simulink library "PhaseCurrentsChecker"  (R2016b)
settings: Solver=VariableStepAuto  StartTime=0.0  StopTime=10.0  RelTol=1e-3
undefined symbols (not defined in the file): maxPhasePeakCurrent
settings Model: Creator=Nathan  LastModifiedBy=march

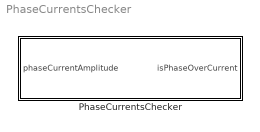
== system PhaseCurrentsChecker ==
  PhaseCurrentsChecker : Subsystem

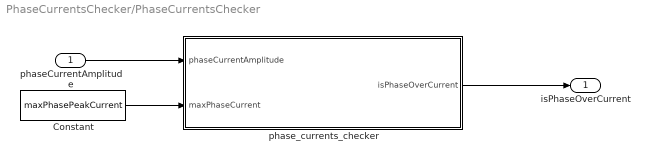
== system PhaseCurrentsChecker/PhaseCurrentsChecker ==
  phaseCurrentAmplitude : Inport  BusOutputAsStruct=on
  Constant : Constant  Value=maxPhasePeakCurrent  VectorParams1D=off  SampleTime=-1
  phase_currents_checker : MATLAB Function  TreatAsAtomicUnit=on
  isPhaseOverCurrent : Outport
  wires:
  phaseCurrentAmplitude/1 -> phase_currents_checker/1(phaseCurrentAmplitude)
  phase_currents_checker/1(isPhaseOverCurrent) -> isPhaseOverCurrent/1
  Constant/1 -> phase_currents_checker/2(maxPhaseCurrent)

== matlab function PhaseCurrentsChecker/phase_currents_checker ==
  data: phaseCurrentAmplitude input; isPhaseOverCurrent output; maxPhaseCurrent input
function isPhaseOverCurrent = phase_currents_checker(phaseCurrentAmplitude,maxPhaseCurrent)
if(phaseCurrentAmplitude >= maxPhaseCurrent)
    isPhaseOverCurrent = 1;
    %Checks if the phase current does not exceed the maximum allowed current    
else
    isPhaseOverCurrent = 0;
end
end
